simulink model "wheelleg_simulator"  (R2024b)
settings: Solver=VariableStepAuto  StartTime=0.0  StopTime=10.0  RelTol=1e-3
values from neighbouring files (symbols this model uses):
  eta_l = 0.2945    [model_sjtu.m]    (also in model_whx.m = 0.3088)
  g = 9.80665    [model_sjtu.m]
  mb = 16.98    [model_sjtu.m]
  ml = 0.86    [model_sjtu.m]
  N = m_p * diff((x + L * sin(theta)), t, 2) + N_M    [model_whx.m]
  Rl = 0.22    [model_sjtu.m]
  Rw = 0.07    [model_sjtu.m]
undefined symbols (not defined in the file or in its folder): X, Y, Z
libraries: sm_lib x77, nesl_utility x34, simulink x6, slpidlib x2
(part 1 of 3)
settings Model: Creator=Ame  LastModifiedBy=Ame

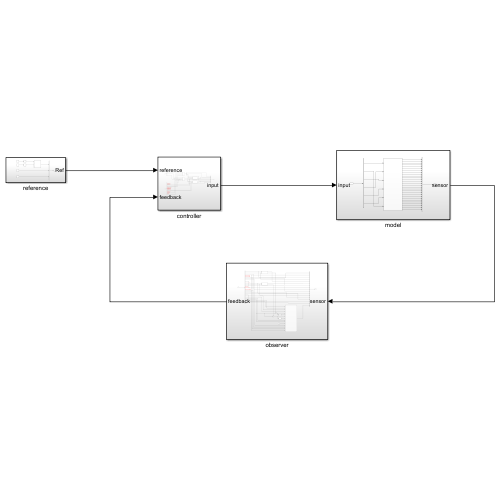
[thumbnail: Simulink's stored preview of the top-level diagram]
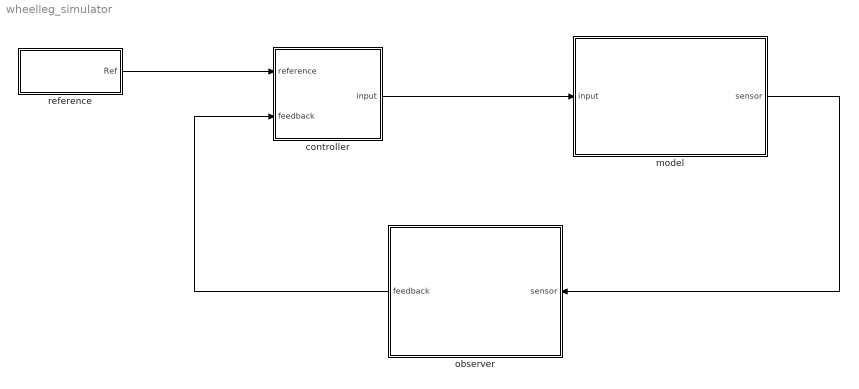
== system wheelleg_simulator ==
  controller : Subsystem
  model : Subsystem
  observer : Subsystem
  reference : Subsystem
  wires:
  model/1(sensor) -> observer/1(sensor)
  reference/1(Ref) -> controller/1(reference)
  observer/1(feedback) -> controller/2(feedback)
  controller/1(input) -> model/1(input)

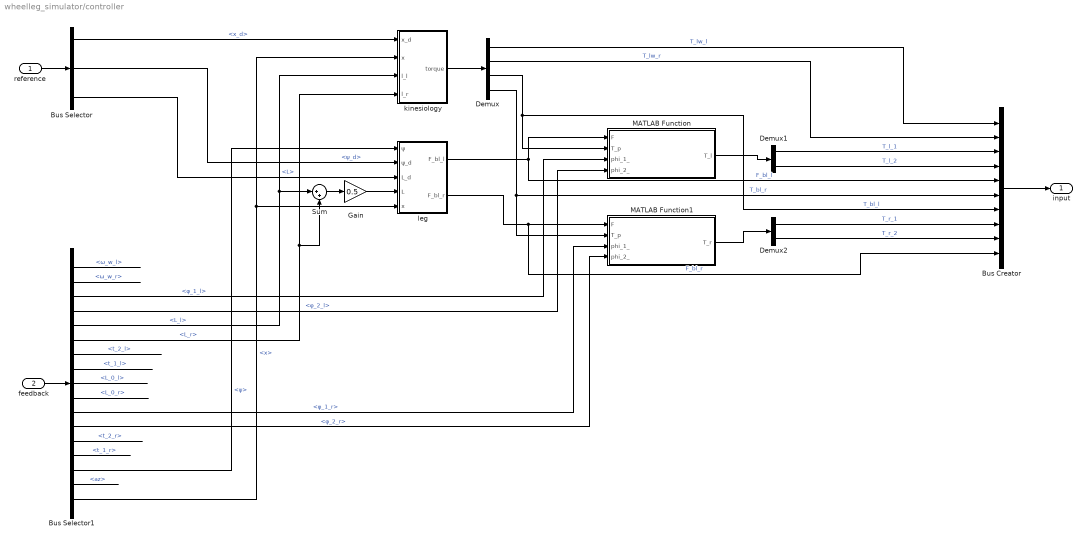
== system wheelleg_simulator/controller ==
  reference : Inport
  feedback : Inport  Port=2
  Bus Creator : BusCreator  Inputs=10
  Bus Selector : BusSelector  OutputSignals=x_d,ψ_d,L
  Bus Selector1 : BusSelector  OutputSignals=ω_w_l,ω_w_r,φ_1_l,φ_2_l,L_l,L_r,t_2_l,t_1_l,L_0_l,L_0_r,φ_1_r,φ_2_r,t_2_r,t_1_r,ψ,az,x
  Demux : Demux
  Demux1 : Demux  Outputs=2
  Demux2 : Demux  Outputs=2
  Gain : Gain  Gain=0.5
  MATLAB Function : MATLAB Function  TreatAsAtomicUnit=on
  MATLAB Function1 : MATLAB Function  TreatAsAtomicUnit=on
  Sum : Sum  Inputs=|++
  "kinesiology " : Subsystem
  leg : Subsystem
  input : Outport
  wires:
  reference/1 -> Bus Selector/1
  Bus Creator/1 -> input/1
  Bus Selector/1 -> "kinesiology "/1(x_d)  "<x_d>"
  Bus Selector/2 -> leg/2(ψ_d)  "<ψ_d>"
  Bus Selector/3 -> leg/3(L_d)  "<L>"
  feedback/1 -> Bus Selector1/1
  Bus Selector1/1 -> ?  "<ω_w_l>"
  Bus Selector1/2 -> ?  "<ω_w_r>"
  Bus Selector1/3 -> MATLAB Function/3(phi_1_)  "<φ_1_l>"
  Bus Selector1/4 -> MATLAB Function/4(phi_2_)  "<φ_2_l>"
  Bus Selector1/5 -> "kinesiology "/3(l_l), Sum/1  "<L_l>"
  Bus Selector1/6 -> Sum/2, "kinesiology "/4(l_r)  "<L_r>"
  Bus Selector1/7 -> ?  "<t_2_l>"
  Bus Selector1/8 -> ?  "<t_1_l>"
  Bus Selector1/9 -> ?  "<L_0_l>"
  Bus Selector1/10 -> ?  "<L_0_r>"
  Bus Selector1/11 -> MATLAB Function1/3(phi_1_)  "<φ_1_r>"
  Bus Selector1/12 -> MATLAB Function1/4(phi_2_)  "<φ_2_r>"
  Bus Selector1/13 -> ?  "<t_2_r>"
  Bus Selector1/14 -> ?  "<t_1_r>"
  Bus Selector1/15 -> leg/1(ψ)  "<ψ>"
  Bus Selector1/16 -> ?  "<az>"
  Bus Selector1/17 -> leg/5(x), "kinesiology "/2(x)  "<x>"
  Sum/1 -> Gain/1
  Gain/1 -> leg/4(L)
  "kinesiology "/1(torque) -> Demux/1
  Demux/1 -> Bus Creator/1  "T_lw_l"
  Demux/2 -> Bus Creator/2  "T_lw_r"
  Demux/3 -> Bus Creator/7, MATLAB Function/2(T_p)  "T_bl_l"
  Demux/4 -> Bus Creator/6, MATLAB Function1/2(T_p)  "T_bl_r"
  leg/1(F_bl_l) -> MATLAB Function/1(F), Bus Creator/5  "F_bl_l"
  leg/2(F_bl_r) -> Bus Creator/10, MATLAB Function1/1(F)  "F_bl_r"
  MATLAB Function/1(T_l) -> Demux1/1
  MATLAB Function1/1(T_r) -> Demux2/1
  Demux1/1 -> Bus Creator/3  "T_l_1"
  Demux1/2 -> Bus Creator/4  "T_l_2"
  Demux2/1 -> Bus Creator/8  "T_r_1"
  Demux2/2 -> Bus Creator/9  "T_r_2"

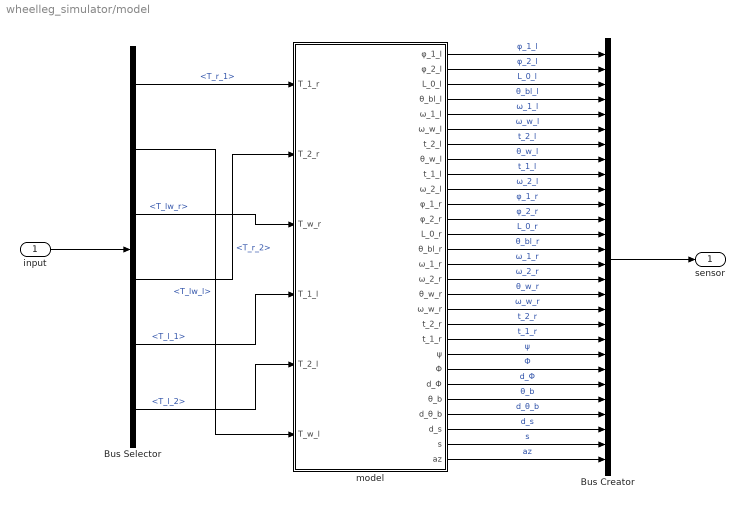
== system wheelleg_simulator/model ==
  input : Inport
  Bus Creator : BusCreator  Inputs=28
  Bus Selector : BusSelector  OutputSignals=T_r_1,T_lw_l,T_lw_r,T_r_2,T_l_1,T_l_2
  model : Subsystem
  sensor : Outport
  wires:
  Bus Creator/1 -> sensor/1
  model/1(φ_1_l) -> Bus Creator/1  "φ_1_l"
  model/2(φ_2_l) -> Bus Creator/2  "φ_2_l"
  model/3(L_0_l) -> Bus Creator/3  "L_0_l"
  model/4(θ_bl_l) -> Bus Creator/4  "θ_bl_l"
  model/5(ω_1_l) -> Bus Creator/5  "ω_1_l"
  model/6(ω_w_l) -> Bus Creator/6  "ω_w_l"
  model/7(t_2_l) -> Bus Creator/7  "t_2_l"
  model/8(θ_w_l) -> Bus Creator/8  "θ_w_l"
  model/10(ω_2_l) -> Bus Creator/10  "ω_2_l"
  model/11(φ_1_r) -> Bus Creator/11  "φ_1_r"
  model/9(t_1_l) -> Bus Creator/9  "t_1_l"
  model/12(φ_2_r) -> Bus Creator/12  "φ_2_r"
  model/13(L_0_r) -> Bus Creator/13  "L_0_r"
  model/14(θ_bl_r) -> Bus Creator/14  "θ_bl_r"
  model/15(ω_1_r) -> Bus Creator/15  "ω_1_r"
  model/16(ω_2_r) -> Bus Creator/16  "ω_2_r"
  model/17(θ_w_r) -> Bus Creator/17  "θ_w_r"
  model/18(ω_w_r) -> Bus Creator/18  "ω_w_r"
  model/20(t_1_r) -> Bus Creator/20  "t_1_r"
  model/19(t_2_r) -> Bus Creator/19  "t_2_r"
  model/21(ψ) -> Bus Creator/21  "ψ"
  model/22(Φ) -> Bus Creator/22  "Φ"
  model/23(d_Φ) -> Bus Creator/23  "d_Φ"
  model/24(θ_b) -> Bus Creator/24  "θ_b"
  model/25(d_θ_b) -> Bus Creator/25  "d_θ_b"
  model/26(d_s) -> Bus Creator/26  "d_s"
  model/27(s) -> Bus Creator/27  "s"
  model/28(az) -> Bus Creator/28  "az"
  input/1 -> Bus Selector/1
  Bus Selector/1 -> model/1(T_1_r)  "<T_r_1>"
  Bus Selector/2 -> model/6(T_w_l)  "<T_lw_l>"
  Bus Selector/3 -> model/3(T_w_r)  "<T_lw_r>"
  Bus Selector/4 -> model/2(T_2_r)  "<T_r_2>"
  Bus Selector/5 -> model/4(T_1_l)  "<T_l_1>"
  Bus Selector/6 -> model/5(T_2_l)  "<T_l_2>"

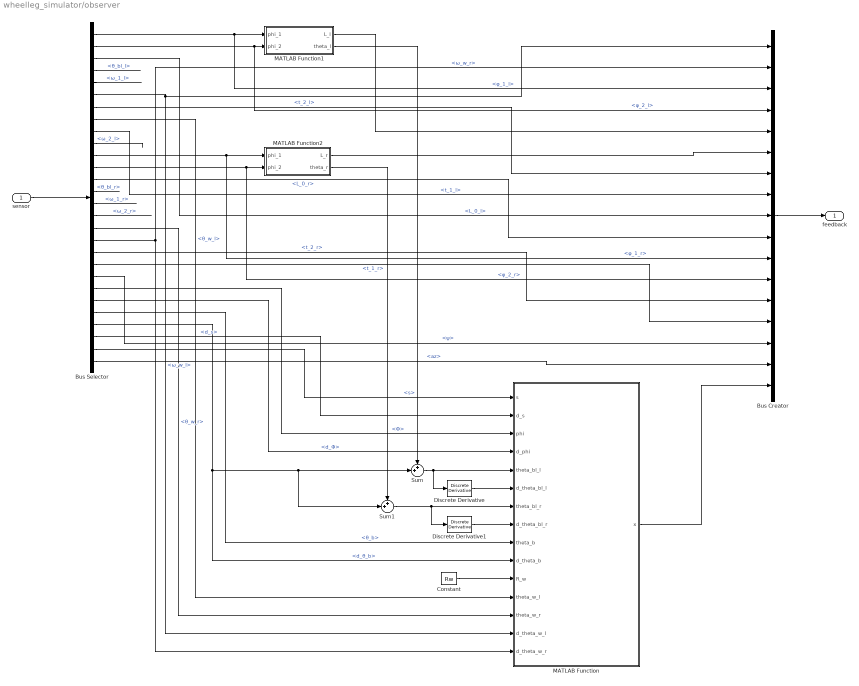
== system wheelleg_simulator/observer ==
  sensor : Inport
  Bus Creator : BusCreator  Inputs=17
  Bus Selector : BusSelector  OutputSignals=φ_1_l,φ_2_l,L_0_l,θ_bl_l,ω_1_l,ω_w_l,t_2_l,θ_w_l,t_1_l,ω_2_l,φ_1_r,φ_2_r,L_0_r,θ_bl_r,ω_1_r,ω_2_r,θ_w_r,ω_w_r,t_2_r,t_1_r,ψ,Φ,d_Φ,θ_b,d_θ_b,d_s,s,az
  Constant : Constant  Value=Rw
  Discrete Derivative : simulink/Discrete/Discrete Derivative  gainval=1.0  ICPrevScaledInput=0.0  OutMin=[]  OutMax=[]  OutDataType=fixdt(1, 16)  OutScaling=2^-10  DoSatur=off
  Discrete Derivative1 : simulink/Discrete/Discrete Derivative  gainval=1.0  ICPrevScaledInput=0.0  OutMin=[]  OutMax=[]  OutDataType=fixdt(1, 16)  OutScaling=2^-10  DoSatur=off
  MATLAB Function : MATLAB Function  TreatAsAtomicUnit=on
  MATLAB Function1 : MATLAB Function  TreatAsAtomicUnit=on
  MATLAB Function2 : MATLAB Function  TreatAsAtomicUnit=on
  Sum : Sum  Inputs=++|
  Sum1 : Sum  Inputs=++|
  feedback : Outport
  wires:
  sensor/1 -> Bus Selector/1
  Bus Selector/16 -> ?  "<ω_2_r>"
  Bus Creator/1 -> feedback/1
  Discrete Derivative1/1 -> MATLAB Function/8(d_theta_bl_r)
  Bus Selector/5 -> ?  "<ω_1_l>"
  Bus Selector/10 -> ?  "<ω_2_l>"
  Bus Selector/20 -> Bus Creator/14  "<t_1_r>"
  Bus Selector/7 -> Bus Creator/7  "<t_2_l>"
  Constant/1 -> MATLAB Function/11(R_w)
  Discrete Derivative/1 -> MATLAB Function/6(d_theta_bl_l)
  Bus Selector/17 -> MATLAB Function/13(theta_w_r)  "<θ_w_r>"
  Bus Selector/9 -> Bus Creator/8  "<t_1_l>"
  Bus Selector/26 -> MATLAB Function/2(d_s)  "<d_s>"
  Bus Selector/27 -> MATLAB Function/1(s)  "<s>"
  Bus Selector/28 -> Bus Creator/16  "<az>"
  Bus Selector/25 -> MATLAB Function/10(d_theta_b), Sum1/2, Sum/2  "<d_θ_b>"
  Bus Selector/24 -> MATLAB Function/9(theta_b)  "<θ_b>"
  Bus Selector/23 -> MATLAB Function/4(d_phi)  "<d_Φ>"
  Bus Selector/22 -> MATLAB Function/3(phi)  "<Φ>"
  Bus Selector/19 -> Bus Creator/13  "<t_2_r>"
  Bus Selector/18 -> MATLAB Function/15(d_theta_w_r), Bus Creator/2  "<ω_w_r>"
  Bus Selector/11 -> Bus Creator/11, MATLAB Function2/1(phi_1)  "<φ_1_r>"
  Bus Selector/12 -> Bus Creator/12, MATLAB Function2/2(phi_2)  "<φ_2_r>"
  Bus Selector/8 -> MATLAB Function/12(theta_w_l)  "<θ_w_l>"
  Bus Selector/6 -> Bus Creator/1, MATLAB Function/14(d_theta_w_l)  "<ω_w_l>"
  Bus Selector/3 -> Bus Creator/9  "<L_0_l>"
  Bus Selector/2 -> Bus Creator/4, MATLAB Function1/2(phi_2)  "<φ_2_l>"
  Bus Selector/1 -> Bus Creator/3, MATLAB Function1/1(phi_1)  "<φ_1_l>"
  MATLAB Function1/1(L_l) -> Bus Creator/5
  MATLAB Function2/1(L_r) -> Bus Creator/6
  MATLAB Function/1(x) -> Bus Creator/17
  Bus Selector/21 -> Bus Creator/15  "<ψ>"
  Bus Selector/15 -> ?  "<ω_1_r>"
  Bus Selector/4 -> ?  "<θ_bl_l>"
  Bus Selector/14 -> ?  "<θ_bl_r>"
  Bus Selector/13 -> Bus Creator/10  "<L_0_r>"
  MATLAB Function1/2(theta_l) -> Sum/1
  Sum/1 -> Discrete Derivative/1, MATLAB Function/5(theta_bl_l)
  MATLAB Function2/2(theta_r) -> Sum1/1
  Sum1/1 -> Discrete Derivative1/1, MATLAB Function/7(theta_bl_r)

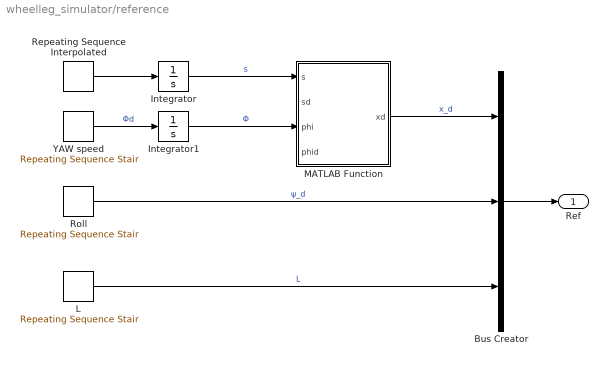
== system wheelleg_simulator/reference ==
  Bus Creator : BusCreator  Inputs=3
  Integrator : Integrator
  Integrator1 : Integrator
  L : simulink/Sources/Repeating Sequence Stair  OutValues=[0.2].'  tsamp=2  OutMin=[]  OutMax=[]  OutDataTypeStr=double  OutputDataTypeScalingMode=double  OutDataType=fixdt(0,8)  ConRadixGroup=Best Precision: Vector-wise  OutScaling=2^-12
  MATLAB Function : MATLAB Function  TreatAsAtomicUnit=on
  Repeating Sequence Interpolated : simulink/Sources/Repeating Sequence Interpolated  OutValues=[0 0 0 0 0 0].'  TimeValues="[0 2 3  4 5 6].'"  LookUpMeth=Interpolation-Use End Values  tsamp=0.001  OutMin=[]  OutMax=[]  OutDataTypeStr=double  OutputDataTypeScalingMode=double  OutDataType=fixdt(0,8)  OutScaling=2^-10
  Roll : simulink/Sources/Repeating Sequence Stair  OutValues=[0].'  tsamp=2  OutMin=[]  OutMax=[]  OutDataTypeStr=double  OutputDataTypeScalingMode=double  OutDataType=fixdt(0,8)  ConRadixGroup=Best Precision: Vector-wise  OutScaling=2^-12
  YAW speed : simulink/Sources/Repeating Sequence Stair  OutValues=[0 ].'  tsamp=2  OutMin=[]  OutMax=[]  OutDataTypeStr=double  OutputDataTypeScalingMode=double  OutDataType=fixdt(0,8)  ConRadixGroup=Best Precision: Vector-wise  OutScaling=2^-12
  Ref : Outport
  wires:
  MATLAB Function/1(xd) -> Bus Creator/1  "x_d"
  L/1 -> Bus Creator/3  "L"
  YAW speed/1 -> Integrator1/1  "Φd"
  Integrator/1 -> MATLAB Function/1(s)  "s"
  Bus Creator/1 -> Ref/1
  Roll/1 -> Bus Creator/2  "ψ_d"
  Repeating Sequence Interpolated/1 -> Integrator/1
  Integrator1/1 -> MATLAB Function/3(phi)  "Φ"

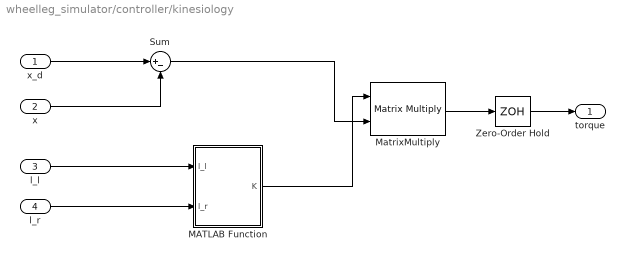
== system wheelleg_simulator/controller/kinesiology  ==
  x_d : Inport
  x : Inport  Port=2
  l_l : Inport  Port=3
  l_r : Inport  Port=4
  MATLAB Function : MATLAB Function  TreatAsAtomicUnit=on
  MatrixMultiply : Product  Multiplication=Matrix(*)
  Sum : Sum  Inputs=|+-
  Zero-Order Hold : ZeroOrderHold  SampleTime=-1
  torque : Outport
  wires:
  l_l/1 -> MATLAB Function/1(l_l)
  l_r/1 -> MATLAB Function/2(l_r)
  x_d/1 -> Sum/1
  x/1 -> Sum/2
  Sum/1 -> MatrixMultiply/2
  MATLAB Function/1(K) -> MatrixMultiply/1
  MatrixMultiply/1 -> Zero-Order Hold/1
  Zero-Order Hold/1 -> torque/1

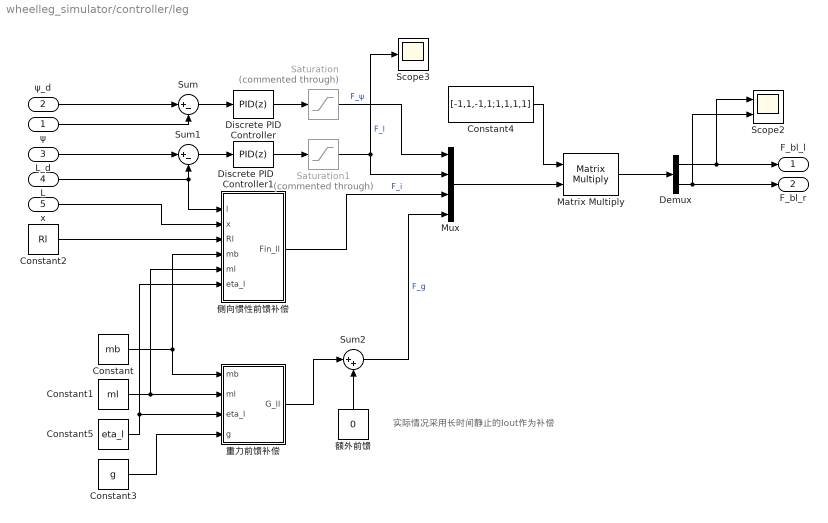
== system wheelleg_simulator/controller/leg ==
  note: 实际情况采用长时间静止的Iout作为补偿
  ψ : Inport
  ψ_d : Inport  Port=2
  L_d : Inport  Port=3
  L : Inport  Port=4
  x : Inport  Port=5
  Constant : Constant  Value=mb
  Constant1 : Constant  Value=ml
  Constant2 : Constant  Value=Rl
  Constant3 : Constant  Value=g
  Constant4 : Constant  Value=[-1,1,-1,1;1,1,1,1]
  Constant5 : Constant  Value=eta_l
  Demux : Demux  Outputs=2
  Discrete PID Controller : slpidlib/PID Controller  Controller=PID  Form=Parallel  TimeDomain=Discrete-time  UseExternalTs=off  SampleTime=0.001  IntegratorMethod=Forward Euler  FilterMethod=Forward Euler  ControllerParametersSource=internal  P=500  I=0  UseKiTs=off  D=10  UseExternalDerivativeSource=off  N=100  UseFilter=off  TunerSelectOption=Transfer Function Based (PID Tuner App)  InitialConditionSource=internal  InitialConditionForIntegrator=0  InitialConditionForFilter=0  DifferentiatorICPrevScaledInput=0  ExternalReset=none  TrackingMode=off  Kt=1  LimitOutput=off  SatLimitsSource=internal  UpperSaturationLimit=inf  LowerSaturationLimit=-inf  LinearizeAsGain=off  AntiWindupMode=none  Kb=1  LimitIntegrator=off  UpperIntegratorSaturationLimit=inf  LowerIntegratorSaturationLimit=-inf  POutMin=[]  POutMax=[]  IOutMin=[]  IOutMax=[]  DOutMin=[]  DOutMax=[]  NOutMin=[]  NOutMax=[]  SumOutMin=[]  SumOutMax=[]  SaturationOutMin=[]  SaturationOutMax=[]  PParamMin=[]  PParamMax=[]  IParamMin=[]  IParamMax=[]  DParamMin=[]  DParamMax=[]  NParamMin=[]  NParamMax=[]  KbParamMin=[]  KbParamMax=[]  KtParamMin=[]  KtParamMax=[]  KbOutMin=[]  KbOutMax=[]  KtOutMin=[]  KtOutMax=[]  IntegratorOutMin=[]  IntegratorOutMax=[]  FilterOutMin=[]  FilterOutMax=[]  SumI1OutMin=[]  SumI1OutMax=[]  SumI2OutMin=[]  SumI2OutMax=[]  SumI3OutMin=[]  SumI3OutMax=[]  SumI4OutMin=[]  SumI4OutMax=[]  SumDOutMin=[]  SumDOutMax=[]  DifferentiatorOutMin=[]  DifferentiatorOutMax=[]  FilterDiffOutCoefMin=[]  FilterDiffOutCoefMax=[]  ReciprocalOutMin=[]  ReciprocalOutMax=[]  SumDenOutMin=[]  SumDenOutMax=[]  SumNumOutMin=[]  SumNumOutMax=[]  DivideOutMin=[]  DivideOutMax=[]  UdiffTsProdOutMin=[]  UdiffTsProdOutMax=[]  NTsProdOutMin=[]  NTsProdOutMax=[]  UintegralTsProdOutMin=[]  UintegralTsProdOutMax=[]  UngainTsProdOutMin=[]  UngainTsProdOutMax=[]  ClampingZeroOutDataTypeStr=Inherit: Inherit via back propagation  ClampingZeroOutMin=[]  ClampingZeroOutMax=[]  FilterDenConstantOutDataTypeStr=Inherit: Inherit via back propagation  FilterDenConstantOutMin=[]  FilterDenConstantOutMax=[]  PCopyOutDataTypeStr=Inherit: Inherit via back propagation  PCopyOutMin=[]  PCopyOutMax=[]  NCopyOutDataTypeStr=Inherit: Inherit via back propagation  NCopyOutMin=[]  NCopyOutMax=[]  IntegratorContinuousStateAttributes=''  IntegratorStateMustResolveToSignalObject=off  IntegratorRTWStateStorageClass=Auto  FilterContinuousStateAttributes=''  FilterStateMustResolveToSignalObject=off  FilterRTWStateStorageClass=Auto  ParallelPVariant=InternalParameters  IdealPVariant=Disabled  IVariant=InternalParameters  DVariant=InternalParameters  IntegratorVariant=Discrete  SatVariant=Disabled  AWVariant=Passthrough  PCopyVariant=Disabled  TRVariant=Disabled  FdbkBlocksVariant=Forward  IdealPFdbkVariant=Disabled  SatFdbkVariant=Disabled  DerivativeFilterVariant=Differentiator  NVariant=Passthrough  NCopyVariant=Disabled_SignalSpec  FilterICVariant=InternalICsDifferentiator  IntegratorICVariant=InternalICs  ExternalResetVariant=Disabled  TRSumVariant=Passthrough  SumFdbkVariant=Disabled  SumVariant=Sum_PID  TsampFilterVariant=InternalTs  TsampNgainVariant=Passthrough  TsampIntegralVariant=Disabled_SignalSpec  ExternalSaturationOutDataTypeStr=Inherit: Same as second input  DerivativeSourceVariant=ErrorSignal  PreIntVariant=InternalPreInt
      settings: LibrarySourceBlock=simulink/Discrete/Discrete PID Controller
  Discrete PID Controller1 : slpidlib/PID Controller  Controller=PID  Form=Parallel  TimeDomain=Discrete-time  UseExternalTs=off  SampleTime=0.001  IntegratorMethod=Forward Euler  FilterMethod=Forward Euler  ControllerParametersSource=internal  P=1500  I=0  UseKiTs=off  D=200  UseExternalDerivativeSource=off  N=100  UseFilter=off  TunerSelectOption=Transfer Function Based (PID Tuner App)  InitialConditionSource=internal  InitialConditionForIntegrator=0  InitialConditionForFilter=0  DifferentiatorICPrevScaledInput=0  ExternalReset=none  TrackingMode=off  Kt=1  LimitOutput=off  SatLimitsSource=internal  UpperSaturationLimit=inf  LowerSaturationLimit=-inf  LinearizeAsGain=off  AntiWindupMode=none  Kb=1  LimitIntegrator=off  UpperIntegratorSaturationLimit=inf  LowerIntegratorSaturationLimit=-inf  POutMin=[]  POutMax=[]  IOutMin=[]  IOutMax=[]  DOutMin=[]  DOutMax=[]  NOutMin=[]  NOutMax=[]  SumOutMin=[]  SumOutMax=[]  SaturationOutMin=[]  SaturationOutMax=[]  PParamMin=[]  PParamMax=[]  IParamMin=[]  IParamMax=[]  DParamMin=[]  DParamMax=[]  NParamMin=[]  NParamMax=[]  KbParamMin=[]  KbParamMax=[]  KtParamMin=[]  KtParamMax=[]  KbOutMin=[]  KbOutMax=[]  KtOutMin=[]  KtOutMax=[]  IntegratorOutMin=[]  IntegratorOutMax=[]  FilterOutMin=[]  FilterOutMax=[]  SumI1OutMin=[]  SumI1OutMax=[]  SumI2OutMin=[]  SumI2OutMax=[]  SumI3OutMin=[]  SumI3OutMax=[]  SumI4OutMin=[]  SumI4OutMax=[]  SumDOutMin=[]  SumDOutMax=[]  DifferentiatorOutMin=[]  DifferentiatorOutMax=[]  FilterDiffOutCoefMin=[]  FilterDiffOutCoefMax=[]  ReciprocalOutMin=[]  ReciprocalOutMax=[]  SumDenOutMin=[]  SumDenOutMax=[]  SumNumOutMin=[]  SumNumOutMax=[]  DivideOutMin=[]  DivideOutMax=[]  UdiffTsProdOutMin=[]  UdiffTsProdOutMax=[]  NTsProdOutMin=[]  NTsProdOutMax=[]  UintegralTsProdOutMin=[]  UintegralTsProdOutMax=[]  UngainTsProdOutMin=[]  UngainTsProdOutMax=[]  ClampingZeroOutDataTypeStr=Inherit: Inherit via back propagation  ClampingZeroOutMin=[]  ClampingZeroOutMax=[]  FilterDenConstantOutDataTypeStr=Inherit: Inherit via back propagation  FilterDenConstantOutMin=[]  FilterDenConstantOutMax=[]  PCopyOutDataTypeStr=Inherit: Inherit via back propagation  PCopyOutMin=[]  PCopyOutMax=[]  NCopyOutDataTypeStr=Inherit: Inherit via back propagation  NCopyOutMin=[]  NCopyOutMax=[]  IntegratorContinuousStateAttributes=''  IntegratorStateMustResolveToSignalObject=off  IntegratorRTWStateStorageClass=Auto  FilterContinuousStateAttributes=''  FilterStateMustResolveToSignalObject=off  FilterRTWStateStorageClass=Auto  ParallelPVariant=InternalParameters  IdealPVariant=Disabled  IVariant=InternalParameters  DVariant=InternalParameters  IntegratorVariant=Discrete  SatVariant=Disabled  AWVariant=Passthrough  PCopyVariant=Disabled  TRVariant=Disabled  FdbkBlocksVariant=Forward  IdealPFdbkVariant=Disabled  SatFdbkVariant=Disabled  DerivativeFilterVariant=Differentiator  NVariant=Passthrough  NCopyVariant=Disabled_SignalSpec  FilterICVariant=InternalICsDifferentiator  IntegratorICVariant=InternalICs  ExternalResetVariant=Disabled  TRSumVariant=Passthrough  SumFdbkVariant=Disabled  SumVariant=Sum_PID  TsampFilterVariant=InternalTs  TsampNgainVariant=Passthrough  TsampIntegralVariant=Disabled_SignalSpec  ExternalSaturationOutDataTypeStr=Inherit: Same as second input  DerivativeSourceVariant=ErrorSignal  PreIntVariant=InternalPreInt
      settings: LibrarySourceBlock=simulink/Discrete/Discrete PID Controller
  Matrix Multiply : Product  Multiplication=Matrix(*)
  Mux : Mux
  Saturation : Saturate  Commented=through
  Saturation1 : Saturate  Commented=through
  Scope2 : Scope  NumInputPorts=2
  Scope3 : Scope
  Sum : Sum  Inputs=|+-
  Sum1 : Sum  Inputs=|+-
  Sum2 : Sum  Inputs=|++
  侧向惯性前馈补偿 : MATLAB Function  TreatAsAtomicUnit=on
  重力前馈补偿 : MATLAB Function  TreatAsAtomicUnit=on
  额外前馈 : Constant  Value=0
  F_bl_l : Outport
  F_bl_r : Outport  Port=2
  wires:
  L/1 -> 侧向惯性前馈补偿/1(l), Sum1/2
  额外前馈/1 -> Sum2/2
  Saturation1/1 -> Mux/2, Scope3/1  "F_l"
  Sum1/1 -> Discrete PID Controller1/1
  重力前馈补偿/1(G_ll) -> Sum2/1
  Constant2/1 -> 侧向惯性前馈补偿/3(Rl)
  Mux/1 -> Matrix Multiply/2
  x/1 -> 侧向惯性前馈补偿/2(x)
  ψ/1 -> Sum/2
  Sum/1 -> Discrete PID Controller/1
  ψ_d/1 -> Sum/1
  Discrete PID Controller1/1 -> Saturation1/1
  侧向惯性前馈补偿/1(Fin_ll) -> Mux/3  "F_i"
  Sum2/1 -> Mux/4  "F_g"
  Constant4/1 -> Matrix Multiply/1
  Demux/2 -> F_bl_r/1, Scope2/2
  Demux/1 -> F_bl_l/1, Scope2/1
  Saturation/1 -> Mux/1  "F_ψ"
  Matrix Multiply/1 -> Demux/1
  Discrete PID Controller/1 -> Saturation/1
  L_d/1 -> Sum1/1
  Constant/1 -> 重力前馈补偿/1(mb), 侧向惯性前馈补偿/4(mb)
  Constant1/1 -> 重力前馈补偿/2(ml), 侧向惯性前馈补偿/5(ml)
  Constant5/1 -> 重力前馈补偿/3(eta_l), 侧向惯性前馈补偿/6(eta_l)
  Constant3/1 -> 重力前馈补偿/4(g)

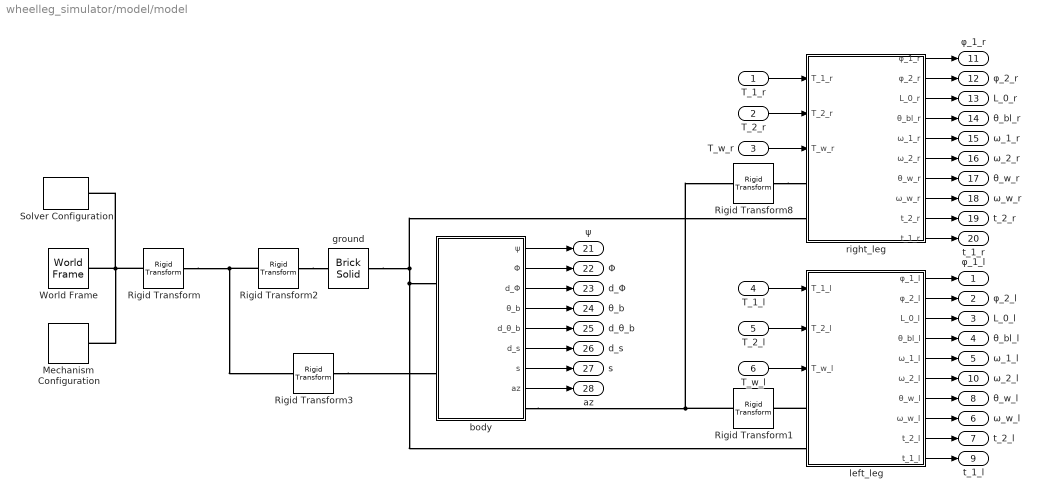
== system wheelleg_simulator/model/model ==
  T_1_r : Inport
  T_2_r : Inport  Port=2
  T_w_r : Inport  Port=3
  T_1_l : Inport  Port=4
  T_2_l : Inport  Port=5
  T_w_l : Inport  Port=6
  Mechanism Configuration : sm_lib/Utilities/Mechanism Configuration  UniformGravity=Constant  GravityVector=[0 0 -9.80665]  GravityVectorUnits=m/s^2  LinearizationDelta=0.001  JointModeTransitionNonlinearIterations=2
  Rigid Transform : sm_lib/Frames and Transforms/Rigid Transform  RotationMethod=StandardAxis  FollAlignAxisA=+X  BaseAlignAxisA=+Y  FollAlignAxisB=+Y  BaseAlignAxisB=+Z  RotationStandardAxis=-X  RotationAngle=90  RotationAngleUnits=deg  RotationArbitraryAxis=[0 0 1]  RotationSequenceAxes=FollowerAxes  RotationSequence=XYX  RotationSequenceAngles=[0 0 0]  RotationSequenceAnglesUnits=deg  RotationMatrix=[1 0 0;0 0 1;0 1 0]  Quaternion=[1 0 0 0]  TranslationMethod=None  TranslationCartesianOffset=[0 0 0]  TranslationCartesianOffsetUnits=m  TranslationStandardAxis=+Z  TranslationStandardOffset=0  TranslationStandardOffsetUnits=m  TranslationROffset=0  TranslationROffsetUnits=m  TranslationThetaOffset=0  TranslationThetaOffsetUnits=deg  TranslationZOffset=0  TranslationZOffsetUnits=m
  Rigid Transform1 : sm_lib/Frames and Transforms/Rigid Transform  RotationMethod=None  FollAlignAxisA=+X  BaseAlignAxisA=+Y  FollAlignAxisB=+Y  BaseAlignAxisB=+Z  RotationStandardAxis=+Z  RotationAngle=0  RotationAngleUnits=deg  RotationArbitraryAxis=[0 0 1]  RotationSequenceAxes=FollowerAxes  RotationSequence=XYX  RotationSequenceAngles=[0 0 0]  RotationSequenceAnglesUnits=deg  RotationMatrix=[1 0 0;0 1 0;0 0 1]  Quaternion=[1 0 0 0]  TranslationMethod=StandardAxis  TranslationCartesianOffset=[0 0 0]  TranslationCartesianOffsetUnits=m  TranslationStandardAxis=+Z  TranslationStandardOffset=0.15  TranslationStandardOffsetUnits=m  TranslationROffset=0  TranslationROffsetUnits=m  TranslationThetaOffset=0  TranslationThetaOffsetUnits=deg  TranslationZOffset=0  TranslationZOffsetUnits=m
  Rigid Transform2 : sm_lib/Frames and Transforms/Rigid Transform  RotationMethod=None  FollAlignAxisA=+X  BaseAlignAxisA=+Y  FollAlignAxisB=+Y  BaseAlignAxisB=+Z  RotationStandardAxis=+Z  RotationAngle=0  RotationAngleUnits=deg  RotationArbitraryAxis=[0 0 1]  RotationSequenceAxes=FollowerAxes  RotationSequence=XYX  RotationSequenceAngles=[0 0 0]  RotationSequenceAnglesUnits=deg  RotationMatrix=[1 0 0;0 1 0;0 0 1]  Quaternion=[1 0 0 0]  TranslationMethod=None  TranslationCartesianOffset=[0 0 0]  TranslationCartesianOffsetUnits=m  TranslationStandardAxis=+Y  TranslationStandardOffset=1  TranslationStandardOffsetUnits=m  TranslationROffset=0  TranslationROffsetUnits=m  TranslationThetaOffset=0  TranslationThetaOffsetUnits=deg  TranslationZOffset=0  TranslationZOffsetUnits=m
  Rigid Transform3 : sm_lib/Frames and Transforms/Rigid Transform  RotationMethod=None  FollAlignAxisA=+X  BaseAlignAxisA=+Y  FollAlignAxisB=+Y  BaseAlignAxisB=+Z  RotationStandardAxis=+Y  RotationAngle=30  RotationAngleUnits=deg  RotationArbitraryAxis=[0 0 1]  RotationSequenceAxes=FollowerAxes  RotationSequence=XYX  RotationSequenceAngles=[0 0 0]  RotationSequenceAnglesUnits=deg  RotationMatrix=[1 0 0;0 0 1;0 1 0]  Quaternion=[1 0 0 0]  TranslationMethod=StandardAxis  TranslationCartesianOffset=[0 0 0]  TranslationCartesianOffsetUnits=m  TranslationStandardAxis=-Y  TranslationStandardOffset=0.35  TranslationStandardOffsetUnits=m  TranslationROffset=0  TranslationROffsetUnits=m  TranslationThetaOffset=0  TranslationThetaOffsetUnits=deg  TranslationZOffset=0  TranslationZOffsetUnits=m
  Rigid Transform8 : sm_lib/Frames and Transforms/Rigid Transform  RotationMethod=None  FollAlignAxisA=+X  BaseAlignAxisA=+Y  FollAlignAxisB=+Y  BaseAlignAxisB=+Z  RotationStandardAxis=+Z  RotationAngle=0  RotationAngleUnits=deg  RotationArbitraryAxis=[0 0 1]  RotationSequenceAxes=FollowerAxes  RotationSequence=XYX  RotationSequenceAngles=[0 0 0]  RotationSequenceAnglesUnits=deg  RotationMatrix=[1 0 0;0 1 0;0 0 1]  Quaternion=[1 0 0 0]  TranslationMethod=StandardAxis  TranslationCartesianOffset=[0 0 0]  TranslationCartesianOffsetUnits=m  TranslationStandardAxis=-Z  TranslationStandardOffset=0.15  TranslationStandardOffsetUnits=m  TranslationROffset=0  TranslationROffsetUnits=m  TranslationThetaOffset=0  TranslationThetaOffsetUnits=deg  TranslationZOffset=0  TranslationZOffsetUnits=m
  Solver Configuration : nesl_utility/Solver Configuration  PhysicalDomain=network_engine_domain  SubClassName=solver  LeftPortType=input  RightPortType=generic  Tones=[]  Harmonics=[]  SimulateNoise=off  Profile=off  UseLocalSampling=off  EnableSwitchedLinearOptims=on  FrequencyDomain=off  UseCCode=off  RelTol=0.001  AbsTol=0.001  MinStep=1e-09  ToWorkspace=off  RevertToSquareIcSolve=off  NumHomotopyIterations=100  PhasorMode=off  PhasorModeNumHarmonics=1  ConsistencySolver=NEWTON_XTOL_AFTER_FTOL  IndexReductionMethod=DerivativeReplacement  DoDC=off  ResidualTolerance=1e-09  ConsistencyTolSource=GLOBAL  ConsistencyAbsTol=0.001  ConsistencyRelTol=0.001  ConsistencyTolFactor=0.001  UseLocalSolver=off  LocalSolverChoice=NE_BACKWARD_EULER_ADVANCER  ResolveIndetEquations=on  FunctionEvalNumThread=1  LocalSolverSampleTime=0.001  DoFixedCost=off  MaxNonlinIter=3  MaxModeIter=2  ComputeImpulses=off  ImpulseIterations=2  LinearAlgebra=auto  LinearAlgebraNumThread=0  EquationFormulation=NE_TIME_EF  DelaysMemoryBudget=1024  AutomaticFiltering=on  FilteringTimeConstant=0.001  PartitionStorageMethod=AS_NEEDED  PartitionMemoryBudget=1024  PartitionMethod=ROBUST  MultibodyUseLocalSolver=off  MultibodyLocalSolverChoice=ODE1  MultibodyLocalSolverSampleTime=0.001
  World Frame : sm_lib/Frames and Transforms/World Frame
  body : Subsystem
  ground : sm_lib/Body Elements/Brick Solid  BrickDimensions=[20 0.1 1]  BrickDimensionsUnits=m  ExportEntireGeometry=on  InertiaType=CalculateFromGeometry  BasedOnType=Density  Density=1000  DensityUnits=kg/m^3  Mass=1  MassUnits=kg  CenterOfMass=[0 0 0]  CenterOfMassUnits=m  MomentsOfInertia=[1 1 1]  MomentsOfInertiaUnits=kg*m^2  ProductsOfInertia=[0 0 0]  ProductsOfInertiaUnits=kg*m^2  GraphicType=FromGeometry  MarkerShape=Sphere  MarkerSize=10  GraphicVisPropType=SimpleVisualProperties  GraphicDiffuseColor=[0.5 0.5 0.5]  GraphicOpacity=1  GraphicSpecularColor=[0.5 0.5 0.5 1.0]  GraphicAmbientColor=[0.15 0.15 0.15 1.0]  GraphicEmissiveColor=[0.0 0.0 0.0 1.0]  GraphicShininess=75  DoExposeReferenceFrame=on  SerializedFrames=<Frames/>
  left_leg : Subsystem
  right_leg : Subsystem
  φ_1_l : Outport
  φ_2_l : Outport  Port=2
  L_0_l : Outport  Port=3
  θ_bl_l : Outport  Port=4
  ω_1_l : Outport  Port=5
  ω_w_l : Outport  Port=6
  t_2_l : Outport  Port=7
  θ_w_l : Outport  Port=8
  t_1_l : Outport  Port=9
  ω_2_l : Outport  Port=10
  φ_1_r : Outport  Port=11
  φ_2_r : Outport  Port=12
  L_0_r : Outport  Port=13
  θ_bl_r : Outport  Port=14
  ω_1_r : Outport  Port=15
  ω_2_r : Outport  Port=16
  θ_w_r : Outport  Port=17
  ω_w_r : Outport  Port=18
  t_2_r : Outport  Port=19
  t_1_r : Outport  Port=20
  ψ : Outport  Port=21
  Φ : Outport  Port=22
  d_Φ : Outport  Port=23
  θ_b : Outport  Port=24
  d_θ_b : Outport  Port=25
  d_s : Outport  Port=26
  s : Outport  Port=27
  az : Outport  Port=28
  wires:
  left_leg/1(φ_1_l) -> φ_1_l/1
  left_leg/5(ω_1_l) -> ω_1_l/1
  left_leg/4(θ_bl_l) -> θ_bl_l/1
  left_leg/3(L_0_l) -> L_0_l/1
  left_leg/2(φ_2_l) -> φ_2_l/1
  left_leg/6(ω_2_l) -> ω_2_l/1
  left_leg/10(t_1_l) -> t_1_l/1
  left_leg/9(t_2_l) -> t_2_l/1
  left_leg/8(ω_w_l) -> ω_w_l/1
  left_leg/7(θ_w_l) -> θ_w_l/1
  right_leg/1(φ_1_r) -> φ_1_r/1
  right_leg/2(φ_2_r) -> φ_2_r/1
  right_leg/7(θ_w_r) -> θ_w_r/1
  right_leg/6(ω_2_r) -> ω_2_r/1
  right_leg/10(t_1_r) -> t_1_r/1
  right_leg/9(t_2_r) -> t_2_r/1
  right_leg/8(ω_w_r) -> ω_w_r/1
  right_leg/5(ω_1_r) -> ω_1_r/1
  right_leg/4(θ_bl_r) -> θ_bl_r/1
  right_leg/3(L_0_r) -> L_0_r/1
  body/1(ψ) -> ψ/1
  body/2(Φ) -> Φ/1
  body/3(d_Φ) -> d_Φ/1
  body/4(θ_b) -> θ_b/1
  body/5(d_θ_b) -> d_θ_b/1
  T_w_r/1 -> right_leg/3(T_w_r)
  T_2_r/1 -> right_leg/2(T_2_r)
  T_1_r/1 -> right_leg/1(T_1_r)
  T_1_l/1 -> left_leg/1(T_1_l)
  T_2_l/1 -> left_leg/2(T_2_l)
  T_w_l/1 -> left_leg/3(T_w_l)
  body/6(d_s) -> d_s/1
  body/7(s) -> s/1
  body/8(az) -> az/1
  connections:
  World Frame/RConn1 -- Rigid Transform/LConn1 -- Solver Configuration/RConn1 -- Mechanism Configuration/RConn1
  left_leg/LConn1 -- Rigid Transform1/RConn1
  Rigid Transform8/RConn1 -- right_leg/LConn1
  Rigid Transform1/LConn1 -- body/RConn1 -- Rigid Transform8/LConn1
  Rigid Transform/RConn1 -- Rigid Transform2/LConn1 -- Rigid Transform3/LConn1
  Rigid Transform2/RConn1 -- ground/RConn1
  Rigid Transform3/RConn1 -- body/LConn2
  ground/LConn1 -- left_leg/LConn2 -- body/LConn1 -- right_leg/LConn2

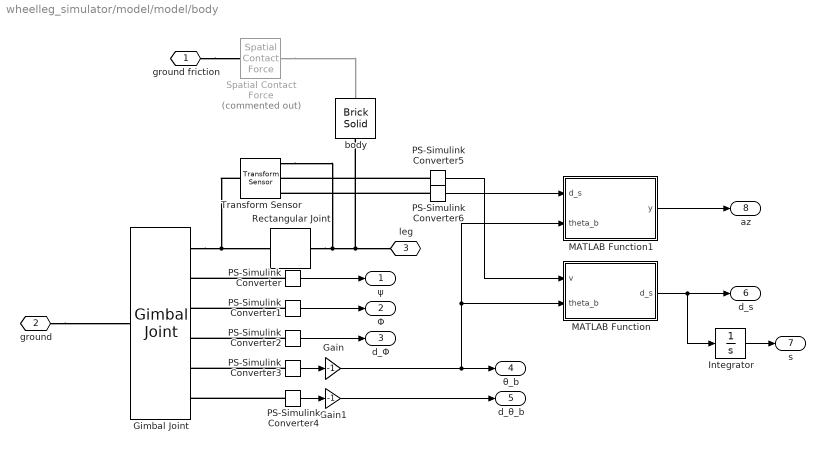
== system wheelleg_simulator/model/model/body ==
  Gain : Gain  Gain=-1
  Gain1 : Gain  Gain=-1
  Gimbal Joint : sm_lib/Joints/Gimbal Joint  JointMode=Normal  CompositeWrenchDir=FollowerOnBase  CompositeWrenchFrame=BaseFrame  SenseConstraintForce=off  SenseConstraintTorque=off  SenseTotalForce=off  SenseTotalTorque=off  RxPositionTargetSpecify=off  RxPositionTargetPriority=High  RxPositionTargetValue=10  RxPositionTargetValueUnits=deg  RxVelocityTargetSpecify=off  RxVelocityTargetPriority=High  RxVelocityTargetValue=0  RxVelocityTargetValueUnits=deg/s  RxEquilibriumPosition=0  RxEquilibriumPositionUnits=deg  RxSpringStiffness=0  RxSpringStiffnessUnits=N*m/deg  RxDampingCoefficient=0  RxDampingCoefficientUnits=N*m/(deg/s)  RxLowerLimitSpecify=off  RxLowerLimitBound=-90  RxLowerLimitBoundUnits=deg  RxLowerLimitStiffness=1e4  RxLowerLimitStiffnessUnits=N*m/deg  RxLowerLimitDamping=10  RxLowerLimitDampingUnits=N*m/(deg/s)  RxLowerLimitTransitionRegionWidth=0.1  RxLowerLimitTransitionRegionWidthUnits=deg  RxUpperLimitSpecify=off  RxUpperLimitBound=90  RxUpperLimitBoundUnits=deg  RxUpperLimitStiffness=1e4  RxUpperLimitStiffnessUnits=N*m/deg  RxUpperLimitDamping=10  RxUpperLimitDampingUnits=N*m/(deg/s)  RxUpperLimitTransitionRegionWidth=0.1  RxUpperLimitTransitionRegionWidthUnits=deg  RxTorqueActuationMode=NoTorque  RxMotionActuationMode=ComputedMotion  RxSensePosition=on  RxSenseVelocity=off  RxSenseAcceleration=off  RxSenseTorqueForce=off  RxSenseLowerLimitTorqueForce=off  RxSenseUpperLimitTorqueForce=off  RyPositionTargetSpecify=off  RyPositionTargetPriority=High  RyPositionTargetValue=45  RyPositionTargetValueUnits=deg  RyVelocityTargetSpecify=off  RyVelocityTargetPriority=High  RyVelocityTargetValue=0  RyVelocityTargetValueUnits=deg/s  RyEquilibriumPosition=0  RyEquilibriumPositionUnits=deg  RySpringStiffness=0  RySpringStiffnessUnits=N*m/deg  RyDampingCoefficient=0  RyDampingCoefficientUnits=N*m/(deg/s)  RyLowerLimitSpecify=off  RyLowerLimitBound=-90  RyLowerLimitBoundUnits=deg  RyLowerLimitStiffness=1e4  RyLowerLimitStiffnessUnits=N*m/deg  RyLowerLimitDamping=10  RyLowerLimitDampingUnits=N*m/(deg/s)  RyLowerLimitTransitionRegionWidth=0.1  RyLowerLimitTransitionRegionWidthUnits=deg  RyUpperLimitSpecify=off  RyUpperLimitBound=90  RyUpperLimitBoundUnits=deg  RyUpperLimitStiffness=1e4  RyUpperLimitStiffnessUnits=N*m/deg  RyUpperLimitDamping=10  RyUpperLimitDampingUnits=N*m/(deg/s)  RyUpperLimitTransitionRegionWidth=0.1  RyUpperLimitTransitionRegionWidthUnits=deg  RyTorqueActuationMode=NoTorque  RyMotionActuationMode=ComputedMotion  RySensePosition=on  RySenseVelocity=on  RySenseAcceleration=off  RySenseTorqueForce=off  RySenseLowerLimitTorqueForce=off  RySenseUpperLimitTorqueForce=off  RzPositionTargetSpecify=on  RzPositionTargetPriority=High  RzPositionTargetValue=-20  RzPositionTargetValueUnits=deg  RzVelocityTargetSpecify=off  RzVelocityTargetPriority=High  RzVelocityTargetValue=0  RzVelocityTargetValueUnits=deg/s  RzEquilibriumPosition=0  RzEquilibriumPositionUnits=deg  RzSpringStiffness=0  RzSpringStiffnessUnits=N*m/deg  RzDampingCoefficient=0  RzDampingCoefficientUnits=N*m/(deg/s)  RzLowerLimitSpecify=off  RzLowerLimitBound=-90  RzLowerLimitBoundUnits=deg  RzLowerLimitStiffness=1e4  RzLowerLimitStiffnessUnits=N*m/deg  RzLowerLimitDamping=10  RzLowerLimitDampingUnits=N*m/(deg/s)  RzLowerLimitTransitionRegionWidth=0.1  RzLowerLimitTransitionRegionWidthUnits=deg  RzUpperLimitSpecify=off  RzUpperLimitBound=90  RzUpperLimitBoundUnits=deg  RzUpperLimitStiffness=1e4  RzUpperLimitStiffnessUnits=N*m/deg  RzUpperLimitDamping=10  RzUpperLimitDampingUnits=N*m/(deg/s)  RzUpperLimitTransitionRegionWidth=0.1  RzUpperLimitTransitionRegionWidthUnits=deg  RzTorqueActuationMode=NoTorque  RzMotionActuationMode=ComputedMotion  RzSensePosition=on  RzSenseVelocity=on  RzSenseAcceleration=off  RzSenseTorqueForce=off  RzSenseLowerLimitTorqueForce=off  RzSenseUpperLimitTorqueForce=off
  Integrator : Integrator
  MATLAB Function : MATLAB Function  TreatAsAtomicUnit=on
  MATLAB Function1 : MATLAB Function  TreatAsAtomicUnit=on
  PS-Simulink Converter{,1..6} (7 alike) : nesl_utility/PS-Simulink Converter  PhysicalDomain=network_engine_domain  SubClassName=ps_output  LeftPortType=input  RightPortType=output  PseudoPeriodic=off  Frequencies=[]  VectorFormat=inherit  Unit=inherit  AffineConversion=off
  Rectangular Joint : sm_lib/Joints/Rectangular Joint  JointMode=Normal  CompositeWrenchDir=FollowerOnBase  CompositeWrenchFrame=BaseFrame  SenseConstraintForce=off  SenseConstraintTorque=off  SenseTotalForce=off  SenseTotalTorque=off  PxPositionTargetSpecify=off  PxPositionTargetPriority=High  PxPositionTargetValue=1  PxPositionTargetValueUnits=m  PxVelocityTargetSpecify=off  PxVelocityTargetPriority=High  PxVelocityTargetValue=0  PxVelocityTargetValueUnits=m/s  PxEquilibriumPosition=0  PxEquilibriumPositionUnits=m  PxSpringStiffness=0  PxSpringStiffnessUnits=N/m  PxDampingCoefficient=0  PxDampingCoefficientUnits=N/(m/s)  PxLowerLimitSpecify=off  PxLowerLimitBound=-1  PxLowerLimitBoundUnits=m  PxLowerLimitStiffness=1e6  PxLowerLimitStiffnessUnits=N/m  PxLowerLimitDamping=1e3  PxLowerLimitDampingUnits=N/(m/s)  PxLowerLimitTransitionRegionWidth=1e-4  PxLowerLimitTransitionRegionWidthUnits=m  PxUpperLimitSpecify=off  PxUpperLimitBound=1  PxUpperLimitBoundUnits=m  PxUpperLimitStiffness=1e6  PxUpperLimitStiffnessUnits=N/m  PxUpperLimitDamping=1e3  PxUpperLimitDampingUnits=N/(m/s)  PxUpperLimitTransitionRegionWidth=1e-4  PxUpperLimitTransitionRegionWidthUnits=m  PxTorqueActuationMode=NoTorque  PxMotionActuationMode=ComputedMotion  PxSensePosition=off  PxSenseVelocity=off  PxSenseAcceleration=off  PxSenseTorqueForce=off  PxSenseLowerLimitTorqueForce=off  PxSenseUpperLimitTorqueForce=off  PyPositionTargetSpecify=off  PyPositionTargetPriority=High  PyPositionTargetValue=0  PyPositionTargetValueUnits=m  PyVelocityTargetSpecify=off  PyVelocityTargetPriority=High  PyVelocityTargetValue=0  PyVelocityTargetValueUnits=m/s  PyEquilibriumPosition=0  PyEquilibriumPositionUnits=m  PySpringStiffness=0  PySpringStiffnessUnits=N/m  PyDampingCoefficient=0  PyDampingCoefficientUnits=N/(m/s)  PyLowerLimitSpecify=off  PyLowerLimitBound=-1  PyLowerLimitBoundUnits=m  PyLowerLimitStiffness=1e6  PyLowerLimitStiffnessUnits=N/m  PyLowerLimitDamping=1e3  PyLowerLimitDampingUnits=N/(m/s)  PyLowerLimitTransitionRegionWidth=1e-4  PyLowerLimitTransitionRegionWidthUnits=m  PyUpperLimitSpecify=off  PyUpperLimitBound=1  PyUpperLimitBoundUnits=m  PyUpperLimitStiffness=1e6  PyUpperLimitStiffnessUnits=N/m  PyUpperLimitDamping=1e3  PyUpperLimitDampingUnits=N/(m/s)  PyUpperLimitTransitionRegionWidth=1e-4  PyUpperLimitTransitionRegionWidthUnits=m  PyTorqueActuationMode=NoTorque  PyMotionActuationMode=ComputedMotion  PySensePosition=off  PySenseVelocity=off  PySenseAcceleration=off  PySenseTorqueForce=off  PySenseLowerLimitTorqueForce=off  PySenseUpperLimitTorqueForce=off
  Spatial Contact Force : sm_lib/Forces and Torques/Spatial Contact Force  Commented=on  NormalForceType=SmoothSpringDamper  NormalStiffness=1e6  NormalStiffnessUnits=N/m  NormalDamping=1e3  NormalDampingUnits=N/(m/s)  NormalTransitionRegionWidth=1e-4  NormalTransitionRegionWidthUnits=m  FrictionType=SmoothStickSlip  CoefficientOfStaticFriction=0.001  CoefficientOfDynamicFriction=0.01  FrictionalCriticalVelocity=1e-3  FrictionalCriticalVelocityUnits=m/s  SenseContactSignal=off  SensePenetrationDepth=off  SenseSeparationDistance=off  SenseNormalForceMagnitude=off  SenseFrictionalForceMagnitude=off  SenseNormalVelocity=off  SenseTangentialVelocity=off  SenseContactBaseRotation=off  SenseContactBaseTranslation=off  SenseContactFollowerRotation=off  SenseContactFollowerTranslation=off  ZeroCrossDetectContactStartAndEnd=off
  Transform Sensor : sm_lib/Frames and Transforms/Transform Sensor  MeasurementFrame=World  RotationSequence=XYX  SenseAngle=off  SenseAxis=off  SenseQ=off  SenseR=off  SenseRotationSequence=off  SenseOmegaX=off  SenseOmegaY=off  SenseOmegaZ=off  SenseOmega=off  SenseQDot=off  SenseRDot=off  SenseRotationSequenceDot=off  SenseAlphaX=off  SenseAlphaY=off  SenseAlphaZ=off  SenseAlpha=off  SenseQDDot=off  SenseRDDot=off  SenseX=off  SenseY=off  SenseZ=off  SenseXYZ=off  SenseRad=off  SenseAzim=off  SenseDist=off  SenseInc=off  SenseXDot=on  SenseYDot=off  SenseZDot=off  SenseXYZDot=off  SenseRadDot=off  SenseAzimDot=off  SenseDistDot=off  SenseIncDot=off  SenseXDDot=off  SenseYDDot=on  SenseZDDot=off  SenseXYZDDot=off  SenseRadDDot=off  SenseAzimDDot=off  SenseDistDDot=off  SenseIncDDot=off
  body : sm_lib/Body Elements/Brick Solid  BrickDimensions=[0.2 0.22 0.30]  BrickDimensionsUnits=m  ExportEntireGeometry=on  InertiaType=CalculateFromGeometry  BasedOnType=Mass  Density=1000  DensityUnits=kg/m^3  Mass=14  MassUnits=kg  CenterOfMass=[0 0 0]  CenterOfMassUnits=m  MomentsOfInertia=[1 1 1]  MomentsOfInertiaUnits=kg*m^2  ProductsOfInertia=[0 0 0]  ProductsOfInertiaUnits=kg*m^2  GraphicType=FromGeometry  MarkerShape=Sphere  MarkerSize=10  GraphicVisPropType=SimpleVisualProperties  GraphicDiffuseColor=[0.5 0.5 0.5]  GraphicOpacity=1  GraphicSpecularColor=[0.5 0.5 0.5 1.0]  GraphicAmbientColor=[0.15 0.15 0.15 1.0]  GraphicEmissiveColor=[0.0 0.0 0.0 1.0]  GraphicShininess=75  DoExposeReferenceFrame=on  SerializedFrames=<Frames/>
  ground friction : PMIOPort  Side=Left
  ground : PMIOPort  Port=2  Side=Left
  leg : PMIOPort  Port=3  Side=Right
  ψ : Outport
  Φ : Outport  Port=2
  d_Φ : Outport  Port=3
  θ_b : Outport  Port=4
  d_θ_b : Outport  Port=5
  d_s : Outport  Port=6
  s : Outport  Port=7
  az : Outport  Port=8
  wires:
  PS-Simulink Converter/1 -> ψ/1
  PS-Simulink Converter1/1 -> Φ/1
  PS-Simulink Converter2/1 -> d_Φ/1
  PS-Simulink Converter3/1 -> Gain/1
  PS-Simulink Converter4/1 -> Gain1/1
  Gain/1 -> MATLAB Function1/2(theta_b), MATLAB Function/2(theta_b), θ_b/1
  Gain1/1 -> d_θ_b/1
  PS-Simulink Converter5/1 -> MATLAB Function/1(v)
  PS-Simulink Converter6/1 -> MATLAB Function1/1(d_s)
  MATLAB Function/1(d_s) -> Integrator/1, d_s/1
  Integrator/1 -> s/1
  MATLAB Function1/1(y) -> az/1
  connections:
  Rectangular Joint/RConn1 -- Transform Sensor/RConn1 -- body/RConn1 -- leg/RConn1
  ground/RConn1 -- Gimbal Joint/LConn1
  Gimbal Joint/RConn1 -- Transform Sensor/LConn1 -- Rectangular Joint/LConn1
  Spatial Contact Force/RConn1 -- body/LConn1
  ground friction/RConn1 -- Spatial Contact Force/LConn1
  PS-Simulink Converter/LConn1 -- Gimbal Joint/RConn2
  PS-Simulink Converter1/LConn1 -- Gimbal Joint/RConn3
  PS-Simulink Converter2/LConn1 -- Gimbal Joint/RConn4
  PS-Simulink Converter3/LConn1 -- Gimbal Joint/RConn5
  PS-Simulink Converter4/LConn1 -- Gimbal Joint/RConn6
  PS-Simulink Converter5/LConn1 -- Transform Sensor/RConn2
  PS-Simulink Converter6/LConn1 -- Transform Sensor/RConn3
